simulink model "doc_fixpt_vitharddec"  (R2014a)
settings: Solver=FixedStepDiscrete  SolverMode=SingleTasking  StartTime=0.0  StopTime=inf  RelTol=1e-3
PreLoadFcn:
  | maxNumErrs = 100;
  | maxNumBits = 1e6;
  | EbNo = 4;
undefined symbols (not defined in the file or in its folder): commblksprivate, Info
libraries: commdigbbndpm3 x2, commcnvcod2 x2, commchan3 x1, commsink2 x1, commrandsrc2 x1
settings Model: MinMaxOverflowLogging=MinMaxAndOverflow  Creator=The MathWorks Inc.
settings DataIOCC: SignalLoggingSaveFormat=ModelDataLogs  SignalLogging=off  SaveTime=off
settings OptimizationCC: InlineParams=on  ExpressionDepthLimit=2147483647  LocalBlockOutputs=off  InitFltsAndDblsToZero=on  OptimizeModelRefInitCode=on  LifeSpan=1
settings DebuggingCC: SaveWithParameterizedLinksMsg=none  UnderspecifiedInitializationDetection=Classic  SignalResolutionControl=TryResolveAllWithWarning  MultiTaskDSMMsg=warning  MultiTaskCondExecSysMsg=none  FcnCallInpInsideContextMsg=UseLocalSettings  StateNameClashWarn=warning  StrictBusMsg=Warning
settings HardwareCC: ProdBitPerInt=16  ProdIntDivRoundTo=Floor  ProdEndianess=LittleEndian  ProdWordSize=16  ProdHWDeviceType=16-bit Generic  TargetBitPerLong=64  TargetBitPerPointer=64  TargetLongLongMode=on  TargetEndianess=LittleEndian  TargetWordSize=64  TargetHWDeviceType=MATLAB Host  ProdEqTarget=off
settings RTWCC: SystemTargetFile=ert.tlc  TemplateMakefile=ert_default_tmf  Description=Real-Time Workshop Embedded Coder (no auto configuration)  GenerateReport=on  RetainRTWFile=on  ProcessScript=ert_make_rtw_hook  IncludeHyperlinkInReport=on  LaunchReport=on  IncludeERTFirstTime=on
settings CodeAppCC: CustomSymbolStrType=$N$R$M  InternalIdentifier=Classic
settings ERTTargetCC: TargetFcnLib=ansi_tfl_tmw.mat  ParMdlRefBuildCompliant=on  CompOptLevelCompliant=on  ConcurrentExecutionCompliant=on  ERTFirstTimeCompliant=on  SupportAbsoluteTime=off  MatFileLogging=on  ModelStepFunctionPrototypeControlCompliant=on  CPPClassGenCompliant=on  ERTCustomFileTemplate=example_file_process.tlc

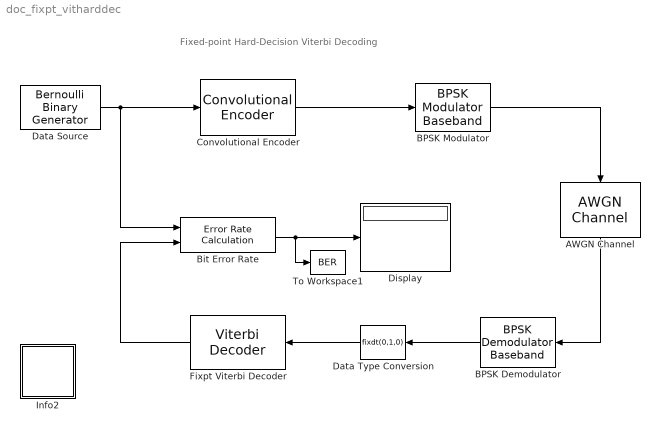
== system doc_fixpt_vitharddec ==
  note: Fixed-point Hard-Decision Viterbi Decoding
  AWGN Channel : commchan3/AWGN Channel  InputProcessing=Columns as channels (frame based)  seed=113  noiseMode="Signal to noise ratio  (Eb/No)"  EbNodB=EbNo - 10*log10(2)  EsNodB=1  SNRdB=10  bitsPerSym=1  Ps=1  Tsym=0.005  variance=1
  BPSK Demodulator : commdigbbndpm3/BPSK Demodulator Baseband  Ph=0  DecType=Hard decision  VarSource=Dialog  Variance=1  outDtype=uint8  derotateFactorWordLen=16
  BPSK Modulator : commdigbbndpm3/BPSK Modulator Baseband  Ph=0  outDtype=double  outWordLen=16  outUDDataType=sfix(16)  outFracLenMode=Best precision  outFracLen=15
  Bit Error Rate : commsink2/Error Rate Calculation  N=56  st_delay=0  cp_mode=Entire frame  subframe=[]  PMode=Port  WsName=ErrorVec  RsMode2=off  stop=on  numErr=maxNumErrs  maxBits=maxNumBits
  Convolutional Encoder : commcnvcod2/Convolutional Encoder  trellis=poly2trellis(9, [561 753])  opMode=Continuous  DelayedResetAction=off  hasIniStPort=off  hasFinStPort=off  usePuncVector=off  punctureVector=[1 1 0 1 1 0].'  reset=Unused parameter value
  Data Source : commrandsrc2/Bernoulli Binary Generator  P=0.5  seed=911  Ts=0.01  frameBased=on  sampPerFrame=100  orient=off  outDataType=boolean
  Data Type Conversion : DataTypeConversion  OutDataTypeStr=fixdt(0,1,0)
  Display : Display
  Fixpt Viterbi Decoder : commcnvcod2/Viterbi Decoder  trellis=poly2trellis(9, [561 753])  isPunctured=off  punctureVector=[1 1 0 1 1 0].'  erasures=off  dectype=Hard decision  runSigValErrCheck=off  nsdecb=3  smWordLength=4  tbdepth=56  opmode=Continuous  reset=off  outDataType=boolean  delayedResetAction=off
  Info2 : Subsystem  AncestorBlock=commblksprivate/Info  mask(Info){}
      settings: OpenFcn=helpview([docroot '/toolbox/comm/comm.map'], 'doc_fixpt_vitharddec')
      mask Display: disp('Info')
  To Workspace1 : ToWorkspace  VariableName=BER  SampleTime=-1
      settings: MaxDataPoints=1
  wires:
  Data Source/1 -> Convolutional Encoder/1, Bit Error Rate/1
  Convolutional Encoder/1 -> BPSK Modulator/1
  BPSK Modulator/1 -> AWGN Channel/1
  AWGN Channel/1 -> BPSK Demodulator/1
  Bit Error Rate/1 -> Display/1, To Workspace1/1
  Fixpt Viterbi Decoder/1 -> Bit Error Rate/2
  BPSK Demodulator/1 -> Data Type Conversion/1
  Data Type Conversion/1 -> Fixpt Viterbi Decoder/1

== system doc_fixpt_vitharddec/Info2 ==
